simulink model "test07"  (R2017a)
settings: Solver=FixedStepAuto  StartTime=0.0  StopTime=4.95  FixedStep=0.05  RelTol=1e-3
undefined symbols (not defined in the file or in its folder): amplitude, delay, widthp
libraries: commchan3 x1
settings Model: Creator=58406  LastModifiedBy=58406

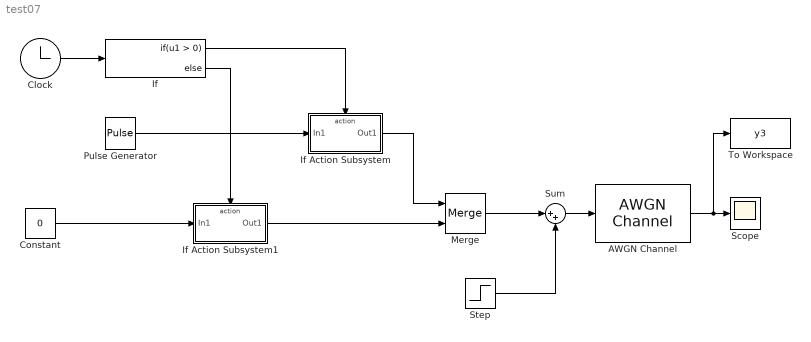
== system test07 ==
  AWGN Channel : commchan3/AWGN Channel  InputProcessing=Columns as channels (frame based)  seed=seed  noiseMode="Signal to noise ratio  (SNR)"  EbNodB=36  EsNodB=10  SNRdB=36  bitsPerSym=1  Ps=1  Tsym=1  variance=1
  Clock : Clock
  Constant : Constant  Value=0
  If : If
  If Action Subsystem : Subsystem  TreatAsAtomicUnit=on
  If Action Subsystem1 : Subsystem  TreatAsAtomicUnit=on
  Merge : Merge
  Pulse Generator : DiscretePulseGenerator  Amplitude=amplitude  Period=1000  PulseWidth=widthp  PhaseDelay=delay  SampleTime=0.05
  Scope : Scope
  Step : Step  Time=0  SampleTime=0.05
  Sum : Sum  Inputs=|++
  To Workspace : ToWorkspace  VariableName=y3  SampleTime=-1
      settings: Save2DSignal=2-D array (concatenate along first dimension)
  wires:
  Clock/1 -> If/1
  If/1 -> If Action Subsystem/Action
  If/2 -> If Action Subsystem1/Action
  Constant/1 -> If Action Subsystem1/1(In1)
  If Action Subsystem/1(Out1) -> Merge/1
  If Action Subsystem1/1(Out1) -> Merge/2
  Pulse Generator/1 -> If Action Subsystem/1(In1)
  Merge/1 -> Sum/1
  Step/1 -> Sum/2
  Sum/1 -> AWGN Channel/1
  AWGN Channel/1 -> To Workspace/1, Scope/1

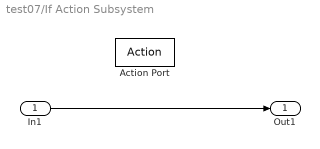
== system test07/If Action Subsystem ==
  In1 : Inport
  Action Port : ActionPort  ActionType=then
  Out1 : Outport
  wires:
  In1/1 -> Out1/1

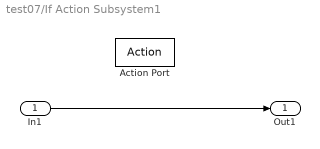
== system test07/If Action Subsystem1 ==
  In1 : Inport
  Action Port : ActionPort  ActionType=else
  Out1 : Outport
  wires:
  In1/1 -> Out1/1
